simulink model "stateflow6"  (R2015a)
settings: Solver=ode3  StartTime=0.0  StopTime=7  RelTol=1e-3
undefined symbols (not defined in the file): ObjLength, ParkLength
libraries: legoev3lib x3
settings Model: SimulationMode=external  ExtModeTrigDuration=2  Creator=Keshav  LastModifiedBy=USER
settings OptimizationCC: OptimizeModelRefInitCode=on  LifeSpan=1
settings DebuggingCC: UnderspecifiedInitializationDetection=Classic  MergeDetectMultiDrivingBlocksExec=none
settings HardwareCC: ProdLargestAtomicInteger=Long  ProdLargestAtomicFloat=Float  ProdEndianess=LittleEndian  ProdHWDeviceType=ARM Compatible->ARM 9
settings RTWCC: SystemTargetFile=realtime.tlc  GenerateMakefile=off  TemplateMakefile=realtime.tmf  Description=Run on Target Hardware  RTWVerbose=off
settings ERTTargetCC: CombineOutputUpdateFcns=off  ERTSrcFileBannerTemplate=realtime_code_template.cgt  ERTHdrFileBannerTemplate=realtime_code_template.cgt  ERTDataSrcFileTemplate=realtime_code_template.cgt  ERTDataHdrFileTemplate=realtime_code_template.cgt  ERTCustomFileTemplate=realtime_file_process.tlc

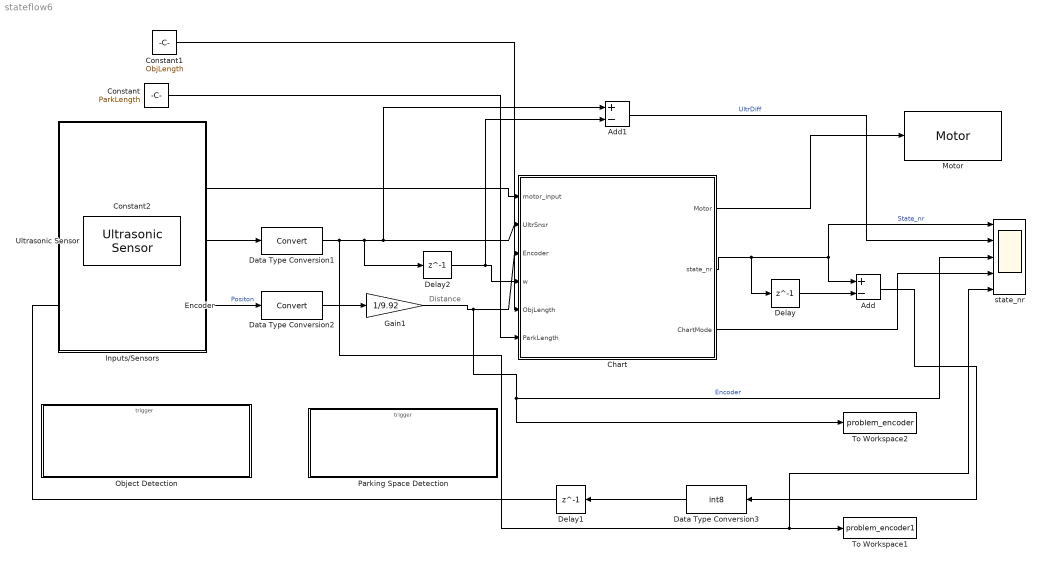
== system stateflow6 ==
  note: Distance
  Add : Sum  Inputs=+-
  Add1 : Sum  Inputs=+-
  Chart : Stateflow chart  TreatAsAtomicUnit=on
  Constant : Constant  Value=ParkLength
  Constant1 : Constant  Value=ObjLength
  Constant2 : Constant  Value=30
  Data Type Conversion1 : DataTypeConversion
  Data Type Conversion2 : DataTypeConversion
  Data Type Conversion3 : DataTypeConversion  OutDataTypeStr=int8
  Delay : Delay  DelayLength=1  InitialCondition=0
  Delay1 : Delay  DelayLength=1  InitialCondition=0
  Delay2 : Delay  DelayLength=1  InitialCondition=0
  Encoder : legoev3lib/Encoder  portNumber=A  opMode=Reset by external signal  sampleTime=0.01
  Gain1 : Gain  Gain=1/9.92
  Inputs/Sensors : Subsystem
  Motor : legoev3lib/Motor  sportNumber=A  sstopAction=Brake
  Object Detection : Subsystem  TreatAsAtomicUnit=on
  Parking Space Detection : Subsystem  TreatAsAtomicUnit=on
  To Workspace1 : ToWorkspace  VariableName=problem_encoder1  SampleTime=-1
  To Workspace2 : ToWorkspace  VariableName=problem_encoder  SampleTime=-1
  Ultrasonic Sensor : legoev3lib/Ultrasonic Sensor  PortNumber=1  sampleTime=0.01
  state_nr : Scope  NumInputPorts=5
      settings: YMin=1~-20~0~1~0  YMax=2~20~300~2~35  SaveName=ScopeData4
  wires:
  Ultrasonic Sensor/1 -> Data Type Conversion1/1
  Data Type Conversion2/1 -> Gain1/1
  Data Type Conversion1/1 -> state_nr/5, To Workspace1/1, Delay2/1, Add1/1, Chart/2(UltrSnsr)
  Constant2/1 -> Chart/1(motor_input)
  Chart/1(Motor) -> Motor/1
  Encoder/1 -> Data Type Conversion2/1  "Positon"
  Gain1/1 -> Chart/3(Encoder), state_nr/3, To Workspace2/1  "Encoder"
  Chart/2(state_nr) -> Delay/1, Add/1, state_nr/1  "State_nr"
  Delay/1 -> Add/2
  Add/1 -> Data Type Conversion3/1
  Data Type Conversion3/1 -> Delay1/1
  Delay1/1 -> Encoder/1
  Chart/3(ChartMode) -> state_nr/4
  Delay2/1 -> Add1/2, Chart/4(w)
  Add1/1 -> state_nr/2  "UltrDiff"
  Constant1/1 -> Chart/5(ObjLength)
  Constant/1 -> Chart/6(ParkLength)

== system stateflow6/Inputs//Sensors ==

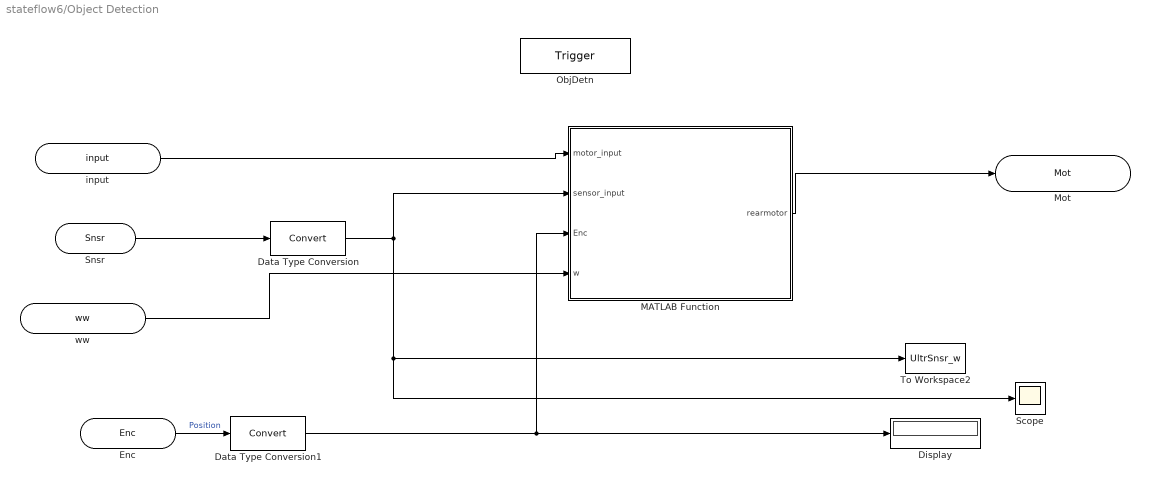
== system stateflow6/Object Detection ==
  ObjDetn : TriggerPort  TriggerType=function-call  IsSimulinkFunction=on  FunctionName=ObjDetn
  Data Type Conversion : DataTypeConversion
  Data Type Conversion1 : DataTypeConversion
  Display : Display
  MATLAB Function : MATLAB Function  TreatAsAtomicUnit=on
  Scope : Scope
      settings: YMin=2.85  YMax=3.15
  To Workspace2 : ToWorkspace  VariableName=UltrSnsr_w  SampleTime=-1
  input : ArgIn  DisableCoverage=on  ArgumentName=input
  Snsr : ArgIn  DisableCoverage=on  Port=2  ArgumentName=Snsr
  Enc : ArgIn  DisableCoverage=on  Port=3  ArgumentName=Enc
  ww : ArgIn  DisableCoverage=on  Port=4  ArgumentName=ww
  Mot : ArgOut  DisableCoverage=on  ArgumentName=Mot
  wires:
  Data Type Conversion/1 -> To Workspace2/1, Scope/1, MATLAB Function/2(sensor_input)
  MATLAB Function/1(rearmotor) -> Mot/1
  Enc/1 -> Data Type Conversion1/1  "Position"
  Snsr/1 -> Data Type Conversion/1
  input/1 -> MATLAB Function/1(motor_input)
  Data Type Conversion1/1 -> Display/1, MATLAB Function/3(Enc)
  ww/1 -> MATLAB Function/4(w)

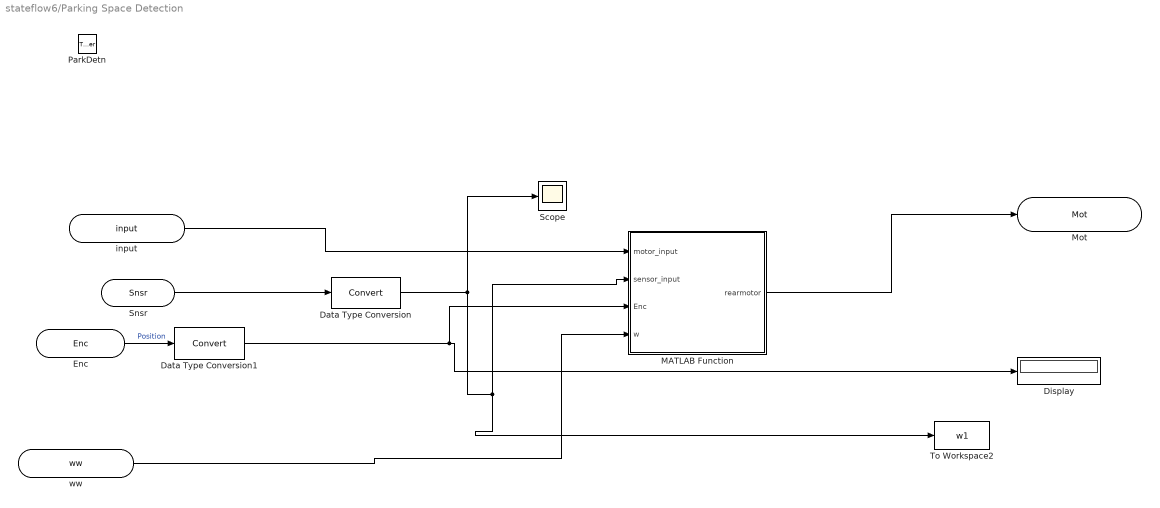
== system stateflow6/Parking Space Detection ==
  ParkDetn : TriggerPort  TriggerType=function-call  IsSimulinkFunction=on  FunctionName=ParkDetn
  Data Type Conversion : DataTypeConversion
  Data Type Conversion1 : DataTypeConversion
  Display : Display
  MATLAB Function : MATLAB Function  TreatAsAtomicUnit=on
  Scope : Scope
      settings: YMin=3  YMax=3
  To Workspace2 : ToWorkspace  VariableName=w1  SampleTime=-1
  input : ArgIn  DisableCoverage=on  ArgumentName=input
  Snsr : ArgIn  DisableCoverage=on  Port=2  ArgumentName=Snsr
  Enc : ArgIn  DisableCoverage=on  Port=3  ArgumentName=Enc
  ww : ArgIn  DisableCoverage=on  Port=4  ArgumentName=ww
  Mot : ArgOut  DisableCoverage=on  ArgumentName=Mot
  wires:
  Data Type Conversion/1 -> To Workspace2/1, MATLAB Function/2(sensor_input), Scope/1
  MATLAB Function/1(rearmotor) -> Mot/1
  Enc/1 -> Data Type Conversion1/1  "Position"
  Snsr/1 -> Data Type Conversion/1
  input/1 -> MATLAB Function/1(motor_input)
  Data Type Conversion1/1 -> MATLAB Function/3(Enc), Display/1
  ww/1 -> MATLAB Function/4(w)

== matlab function stateflow6/Parking Space Detection/MATLAB Function ==
  data: motor_input input; sensor_input input; Enc input; rearmotor output; w input
function rearmotor = fcn(motor_input,sensor_input,Enc,w)
%#codegen
%d = z
%u = 0; %Encoder reset
% x = w;
% length2=0;
%reset11=0;
%state3=0;
if(sensor_input>24)&&(sensor_input<=60)
    rearmotor=motor_input-15;
%     if((sensor_input-w)>2)||((sensor_input-w)<-2)
%         rearmotor = motor_input - 15;
%     elseif(sensor_input>4)&&(sensor_input<=20)
%         rearmotor = motor_input-15;
%      end

  %  if (Enc>=73)&&(Enc<=74)
   %     length2=Enc;
 %       rearmotor=0;
%        reset11=1;
    %    state3=1;        
    %end
    %elseif(sensor_input>20)&&(sensor_input<=35)
 %   rearmotor=motor_input;
%else(sensor_input>24)&&(sensor_input<=61)
 %   x = u;
  %  rearmotor=motor_input-10;
   % u=1;    
    %if(sensor_input<=20)
    %    rearmotor=0;   
%else((sensor_input-z)>2)||((sensor_input-z)<-2)
   % rearmotor=0;
else
    rearmotor = motor_input - 10;

%state3=0;
end



end

== matlab function stateflow6/Object Detection/MATLAB Function ==
  data: motor_input input; sensor_input input; rearmotor output; Enc input; w input
function rearmotor = fcn(motor_input,sensor_input,Enc,w)
%#codegen
%d = z
%u = 0; %Encoder reset
%x = w;
%lenght=0;
%reset1=0;
%state2=0;
if(sensor_input>4)&&(sensor_input<=24)
    rearmotor=motor_input;
%     if((sensor_input-w)>2)|| ((sensor_input-w)<-2)
%         rearmotor = motor_input - 15;
%     elseif(sensor_input>4)&&(sensor_input<=20)
%         rearmotor = motor_input-5;
%     end
%    if (Enc>=30)&&(Enc<=32)
 %       length1=30;
%        rearmotor=0;
%        reset1=1;
     %   state2=1;        
  %  end
    %elseif(sensor_input>20)&&(sensor_input<=35)
 %   rearmotor=motor_input;
%else(sensor_input>24)&&(sensor_input<=61)
 %   x = u;
  %  rearmotor=motor_input-10;
   % u=1;    
    %if(sensor_input<=20)
    %    rearmotor=0;   
%else((sensor_input-z)>2)||((sensor_input-z)<-2)
   % rearmotor=0;
else
    rearmotor = motor_input - 10;
    %state2=0;
end



end

== stateflow chart stateflow6/Chart ==
  state First_Object
    en:
    state_nr=1;
    du:
    Motor = ObjDetn(motor_input,UltrSnsr,Encoder,w);
  state Stop_motor
    entry: Motor=0;
    state_nr=5;
  note: 
  note: 
  state Park_Space
    en:
    state_nr=2;
    du:
    Motor = ParkDetn(motor_input,UltrSnsr,Encoder,w);
    note: 
    note: 
  state Second_Object
    en:
    state_nr=3;
    du:
    Motor = ObjDetn(motor_input,UltrSnsr,Encoder,w);
  (default) -> First_Object
  (junction 160) -> First_Object
  First_Object -> (junction 160) [order 1] : after(200, msec)[(UltrSnsr-w)>2 || (UltrSnsr-w)<-2 && Encoder<ObjLength]
  Second_Object -> (junction 160) [order 1] : after(200, msec)[(UltrSnsr-w)>2 || (UltrSnsr-w)<-2 && Encoder<ObjLength]
  First_Object -> Park_Space [order 2] : [UltrSnsr>24 && Encoder>=ObjLength]
  Park_Space -> First_Object [order 1] : [UltrSnsr<40 && UltrSnsr>24 && Encoder<ParkLength]
  Second_Object -> Stop_motor [order 2] : [UltrSnsr>24 && Encoder>ObjLength]
  Park_Space -> (junction 160) [order 2] : after(200, msec)[(UltrSnsr-w)>2 || (UltrSnsr-w)<-2 && Encoder<ParkLength]
  Park_Space -> Second_Object [order 3] : [UltrSnsr<24 && Encoder>=ParkLength]
  data: motor_input input; Motor output; UltrSnsr input; Encoder input; state_nr output; w input; ChartMode output Enum: ChartModeType; ObjLength input; ParkLength input
